simulink model "Bebop_sim_spline_without_joy"  (R2018a)
settings: Solver=VariableStepAuto  StartTime=0.0  StopTime=15  FixedStep=.05  MaxStep=1  MinStep=0.1  RelTol=200  AbsTol=200
values from neighbouring files (symbols this model uses):
  g = 9.81    [initialize_race_no_realtime.m]    (also in initialize_race_realtime.m; initialize_race_realtime_backup_cubic.m; moving_average_rls_own.m = P(i-1)*meas*(lambda+meas*P(i-1)*meas)^-1)
  gates = sim_gates(:,:,1)    [eval_sim.m]    (also in initialize_race_realtime.m = [dist,0,height,deg2rad(110); initialize_race_realtime_backup_cubic.m = [dist,0,height,deg2rad(110); plot_sim.m)
  max_rot_Z = (90)*pi/180    (= 1.57079632679)    [Bebop_sim_init.m]    (also in initialize_race_no_realtime.m = 1.0471975512; initialize_race_realtime.m; initialize_race_realtime_backup_cubic.m; run_batch1.m = list_agility(idx_agility)*max_rot_Z)
  max_theta_X = (40)*pi/180    (= 0.698131700798)    [Bebop_sim_init.m]    (also in initialize_race_no_realtime.m = 0.13962634016; initialize_race_realtime.m = 1.308996939; initialize_race_realtime_backup_cubic.m = 1.308996939; run_batch1.m = list_agility(idx_agility)*max_theta_X)
  max_theta_Y = (40)*pi/180    (= 0.698131700798)    [Bebop_sim_init.m]    (also in initialize_race_no_realtime.m = 0.13962634016; initialize_race_realtime.m = 1.308996939; initialize_race_realtime_backup_cubic.m = 1.308996939; run_batch1.m = list_agility(idx_agility)*max_theta_Y)
  max_v_Z = .5    (= 0.5)    [Bebop_sim_init.m]    (also in initialize_race_no_realtime.m = 1; initialize_race_realtime.m = 3; initialize_race_realtime_backup_cubic.m = 3; run_batch1.m = list_agility(idx_agility)*max_v_Z)
  splines = zeros(3,4,size(gates,1))    [initialize_race_no_realtime.m]    (also in show_splines.m)
libraries: simulink x4, sharedtransform x2, aerolibutil x1
settings Model: EnablePacing=on  Creator=vinni  LastModifiedBy=vinni
settings HardwareCC: ProdBitPerLong=64  ProdHWDeviceType=Intel->x86-64 (Linux 64)

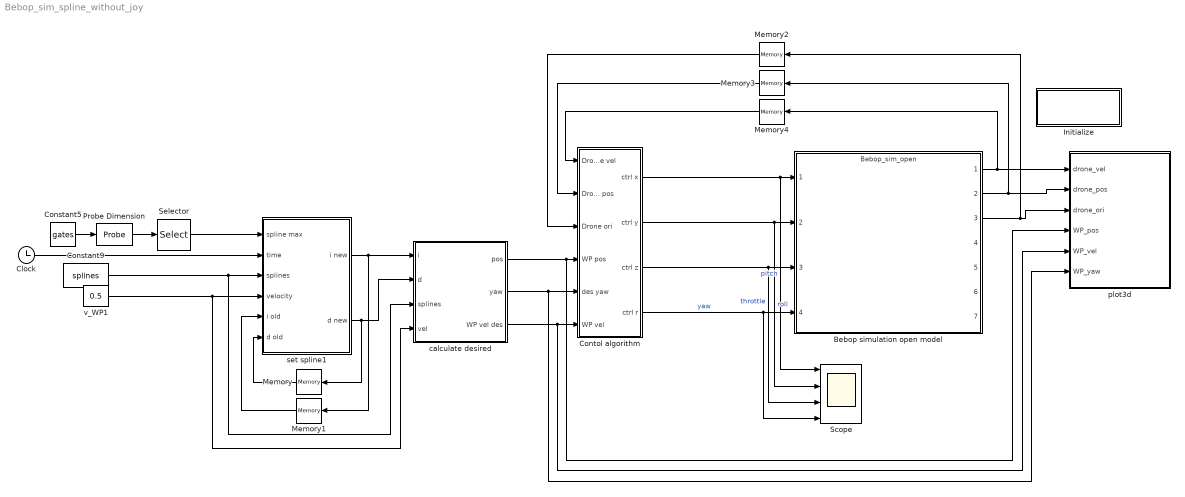
== system Bebop_sim_spline_without_joy ==
  Bebop simulation open model : ModelReference  ModelNameDialog=Bebop_sim_open.slx  SimulationMode=Normal  ModelReferenceVersion=1.31
  Clock : Clock
  Constant5 : Constant  Value=gates
  Constant9 : Constant  Value=splines
  Contol algorithm : Subsystem
  Initialize : Subsystem  TreatAsAtomicUnit=on
  Memory{,1..4} (5 alike) : Memory
  Probe Dimension : Probe  ProbeWidth=off  ProbeSampleTime=off  ProbeComplexSignal=off  ProbeSignalDimensions=on
  Scope : Scope  NumInputPorts=4
  Selector : Selector  IndexOptions=Index vector (dialog)  Indices=1  OutputSizes=1
  calculate desired : Subsystem
  plot3d : MATLAB Function  TreatAsAtomicUnit=on
  set spline1 : Subsystem
  v_WP1 : Constant  Value=0.5  VectorParams1D=off
  wires:
  Bebop simulation open model/2 -> Memory3/1, plot3d/2(drone_pos)
  Bebop simulation open model/3 -> Memory2/1, plot3d/3(drone_ori)
  Contol algorithm/2(ctrl y) -> Scope/2, Bebop simulation open model/2  "roll"
  Bebop simulation open model/1 -> Memory4/1, plot3d/1(drone_vel)
  Contol algorithm/1(ctrl x) -> Scope/1, Bebop simulation open model/1  "pitch"
  Contol algorithm/4(ctrl r) -> Scope/4, Bebop simulation open model/4  "yaw"
  Contol algorithm/3(ctrl z) -> Scope/3, Bebop simulation open model/3  "throttle"
  Constant9/1 -> set spline1/3(splines), calculate desired/3(splines)
  Selector/1 -> set spline1/1(spline max)
  Constant5/1 -> Probe Dimension/1
  Probe Dimension/1 -> Selector/1
  calculate desired/1(pos) -> Contol algorithm/4(WP pos), plot3d/4(WP_pos)
  Clock/1 -> set spline1/2(time)
  calculate desired/2(yaw) -> plot3d/6(WP_yaw), Contol algorithm/5(des yaw)
  calculate desired/3(WP vel des) -> plot3d/5(WP_vel), Contol algorithm/6(WP vel)
  set spline1/2(d new) -> Memory/1, calculate desired/2(d)
  Memory/1 -> set spline1/6(d old)
  set spline1/1(i new) -> Memory1/1, calculate desired/1(i)
  Memory1/1 -> set spline1/5(i old)
  v_WP1/1 -> set spline1/4(velocity), calculate desired/4(vel)
  Memory2/1 -> Contol algorithm/3(Drone ori)
  Memory3/1 -> Contol algorithm/2(Drone pos)
  Memory4/1 -> Contol algorithm/1(Drone vel)

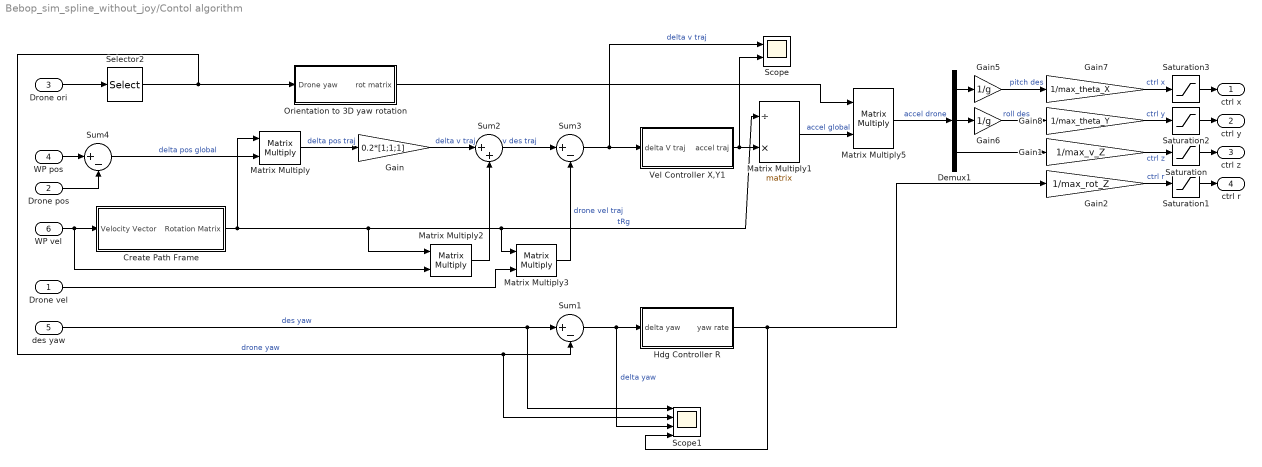
== system Bebop_sim_spline_without_joy/Contol algorithm ==
  Drone vel : Inport
  Drone pos : Inport  Port=2
  Drone ori : Inport  Port=3
  WP pos : Inport  Port=4
  des yaw : Inport  Port=5
  WP vel : Inport  Port=6
  Create Path Frame : Subsystem
  Demux1 : Demux  Outputs=3
  Gain : Gain  Gain=0.2*[1;1;1]
  Gain1 : Gain  Gain=1/max_v_Z
  Gain2 : Gain  Gain=1/max_rot_Z
  Gain5 : Gain  Gain=1/g
  Gain6 : Gain  Gain=1/g
  Gain7 : Gain  Gain=1/max_theta_X
  Gain8 : Gain  Gain=1/max_theta_Y
  Hdg Controller R : Subsystem
  Matrix Multiply{,2..3,5} (4 alike) : Product  Inputs=**  Multiplication=Matrix(*)
  Matrix Multiply1 : Product  Inputs=/*  Multiplication=Matrix(*)
  Orientation to 3D yaw rotation : Subsystem
  Saturation{,1..3} (4 alike) : Saturate  UpperLimit=1  LowerLimit=-1
  Scope : Scope  NumInputPorts=2
  Scope1 : Scope  NumInputPorts=4
  Selector2 : Selector  InputPortWidth=3  IndexOptions=Index vector (dialog)  Indices=3  OutputSizes=1
  Sum1 : Sum  Inputs=|+-
  Sum2 : Sum  Inputs=|++
  Sum3 : Sum  Inputs=|+-
  Sum4 : Sum  Inputs=|+-
  Vel Controller X,Y1 : Subsystem
  ctrl x : Outport
  ctrl y : Outport  Port=2
  ctrl z : Outport  Port=3
  ctrl r : Outport  Port=4
  wires:
  Sum4/1 -> Matrix Multiply/2  "delta pos global"
  Matrix Multiply/1 -> Gain/1  "delta pos traj"
  Create Path Frame/1(Rotation Matrix) -> Matrix Multiply/1, Matrix Multiply2/1, Matrix Multiply1/1, Matrix Multiply3/1  "tRg"
  WP vel/1 -> Matrix Multiply2/2, Create Path Frame/1(Velocity Vector)
  Drone pos/1 -> Sum4/2
  WP pos/1 -> Sum4/1
  Drone vel/1 -> Matrix Multiply3/2
  Gain/1 -> Sum2/1  "delta v traj"
  Drone ori/1 -> Selector2/1
  des yaw/1 -> Scope1/1, Sum1/1  "des yaw"
  Selector2/1 -> Scope1/2, Sum1/2, Orientation to 3D yaw rotation/1(Drone yaw)  "drone yaw"
  Sum1/1 -> Scope1/3, Hdg Controller R/1(delta yaw)  "delta yaw"
  Hdg Controller R/1(yaw rate) -> Scope1/4, Gain2/1
  Sum2/1 -> Sum3/1  "v des traj"
  Matrix Multiply2/1 -> Sum2/2
  Matrix Multiply3/1 -> Sum3/2  "drone vel traj"
  Sum3/1 -> Scope/1, Vel Controller X,Y1/1(delta V traj)  "delta v traj"
  Matrix Multiply1/1 -> Matrix Multiply5/2  "accel global"
  Vel Controller X,Y1/1(accel traj) -> Scope/2, Matrix Multiply1/2
  Orientation to 3D yaw rotation/1(rot matrix) -> Matrix Multiply5/1
  Matrix Multiply5/1 -> Demux1/1  "accel drone"
  Demux1/1 -> Gain5/1
  Demux1/2 -> Gain6/1
  Gain7/1 -> Saturation3/1  "ctrl x"
  Gain8/1 -> Saturation2/1  "ctrl y"
  Saturation2/1 -> ctrl y/1
  Gain5/1 -> Gain7/1  "pitch des"
  Gain6/1 -> Gain8/1  "roll des"
  Saturation3/1 -> ctrl x/1
  Gain1/1 -> Saturation/1  "ctrl z"
  Saturation/1 -> ctrl z/1
  Demux1/3 -> Gain1/1
  Gain2/1 -> Saturation1/1  "ctrl r"
  Saturation1/1 -> ctrl r/1

== system Bebop_sim_spline_without_joy/Initialize ==
  Event Listener : EventListener  DisableCoverage=on  EventName=reset
  reset_plot : MATLAB Function  TreatAsAtomicUnit=on

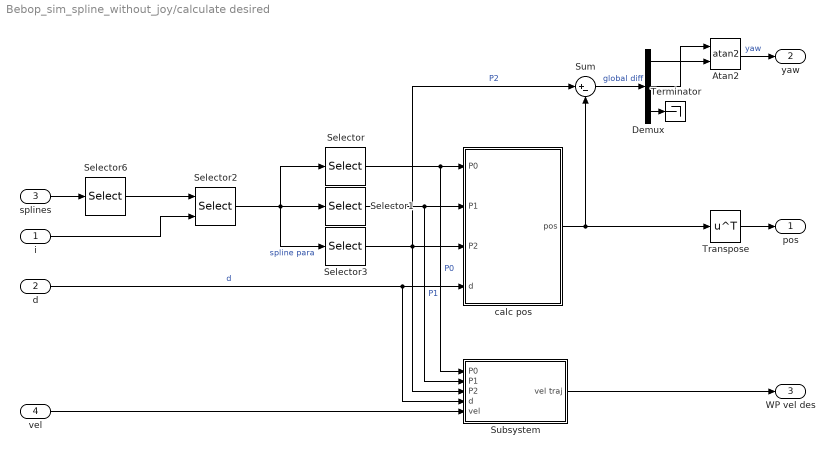
== system Bebop_sim_spline_without_joy/calculate desired ==
  i : Inport
  d : Inport  Port=2
  splines : Inport  Port=3
  vel : Inport  Port=4
  Atan2 : Trigonometry  Operator=atan2
  Demux : Demux  Outputs=3
  Selector : Selector  NumberOfDimensions=2  InputPortWidth=3  IndexOptions=Index vector (dialog),Select all  Indices=1,1  OutputSizes=1,1
  Selector1 : Selector  NumberOfDimensions=2  InputPortWidth=3  IndexOptions=Index vector (dialog),Select all  Indices=2,1  OutputSizes=1,1
  Selector2 : Selector  NumberOfDimensions=3  IndexMode=Zero-based  InputPortWidth=3  IndexOptions=Select all,Select all,Index vector (port)  Indices=3,1,1  OutputSizes=1,1,1
  Selector3 : Selector  NumberOfDimensions=2  InputPortWidth=3  IndexOptions=Index vector (dialog),Select all  Indices=3,1  OutputSizes=1,1
  Selector6 : Selector  NumberOfDimensions=3  InputPortWidth=3  IndexOptions=Select all,Index vector (dialog),Select all  Indices=3,[1,2,3],1  OutputSizes=1,1,1
  Subsystem : Subsystem
  Sum : Sum  Inputs=|+-
  Terminator : Terminator
  Transpose : Math  Operator=transpose  SaturateOnIntegerOverflow=on
  calc pos : Subsystem
  pos : Outport
  yaw : Outport  Port=2
  WP vel des : Outport  Port=3
  wires:
  splines/1 -> Selector6/1
  i/1 -> Selector2/2
  Selector2/1 -> Selector3/1, Selector1/1, Selector/1  "spline para"
  Selector/1 -> Subsystem/1(P0), calc pos/1(P0)  "P0"
  Selector1/1 -> Subsystem/2(P1), calc pos/2(P1)  "P1"
  Selector3/1 -> Sum/1, Subsystem/3(P2), calc pos/3(P2)  "P2"
  d/1 -> calc pos/4(d), Subsystem/4(d)  "d"
  calc pos/1(pos) -> Sum/2, Transpose/1
  Selector6/1 -> Selector2/1
  Sum/1 -> Demux/1  "global diff"
  Demux/2 -> Atan2/1
  Demux/1 -> Atan2/2
  Demux/3 -> Terminator/1
  Atan2/1 -> yaw/1  "yaw"
  vel/1 -> Subsystem/5(vel)
  Subsystem/1(vel traj) -> WP vel des/1
  Transpose/1 -> pos/1

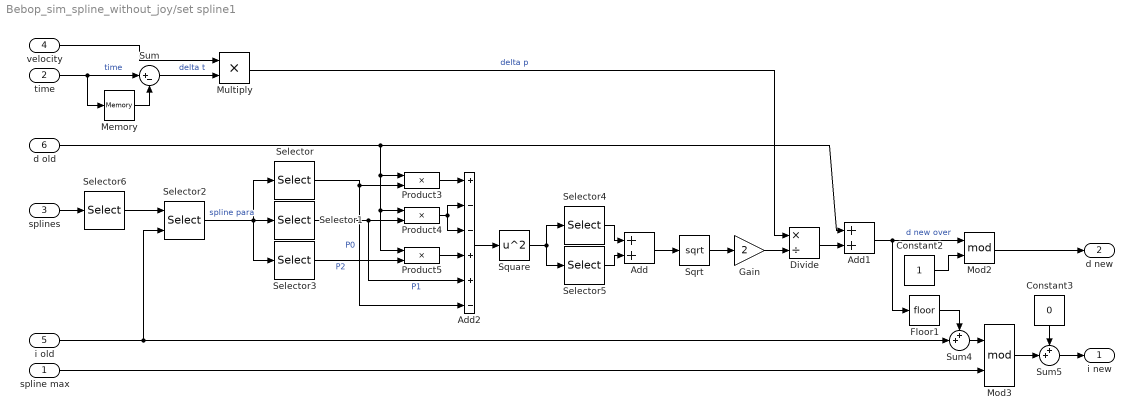
== system Bebop_sim_spline_without_joy/set spline1 ==
  spline max : Inport
  time : Inport  Port=2
  splines : Inport  Port=3
  velocity : Inport  Port=4
  i old : Inport  Port=5
  d old : Inport  Port=6
  Add : Sum
  Add1 : Sum
  Add2 : Sum  Inputs=+--++-
  Constant2 : Constant
  Constant3 : Constant  Value=0
  Divide : Product  Inputs=*/
  Floor1 : Rounding
  Gain : Gain  Gain=2
  Memory : Memory
  Mod2 : Math  Operator=mod  SaturateOnIntegerOverflow=on
  Mod3 : Math  Operator=mod  SaturateOnIntegerOverflow=on
  Multiply : Product
  Product3 : Product
  Product4 : Product
  Product5 : Product
  Selector : Selector  NumberOfDimensions=2  InputPortWidth=3  IndexOptions=Index vector (dialog),Select all  Indices=1,1  OutputSizes=1,1
  Selector1 : Selector  NumberOfDimensions=2  InputPortWidth=3  IndexOptions=Index vector (dialog),Select all  Indices=2,1  OutputSizes=1,1
  Selector2 : Selector  NumberOfDimensions=3  IndexMode=Zero-based  InputPortWidth=3  IndexOptions=Select all,Select all,Index vector (port)  Indices=3,1,1  OutputSizes=1,1,1
  Selector3 : Selector  NumberOfDimensions=2  InputPortWidth=3  IndexOptions=Index vector (dialog),Select all  Indices=3,1  OutputSizes=1,1
  Selector4 : Selector  InputPortWidth=3  IndexOptions=Index vector (dialog)  Indices=2  OutputSizes=1
  Selector5 : Selector  InputPortWidth=3  IndexOptions=Index vector (dialog)  Indices=1  OutputSizes=1
  Selector6 : Selector  NumberOfDimensions=3  InputPortWidth=3  IndexOptions=Select all,Index vector (dialog),Select all  Indices=3,[1,2,3],1  OutputSizes=1,1,1
  Sqrt : Sqrt  SaturateOnIntegerOverflow=on
  Square : Math  Operator=square  SaturateOnIntegerOverflow=on
  Sum : Sum  Inputs=|+-
  Sum4 : Sum  Inputs=++|
  Sum5 : Sum  Inputs=++|
  i new : Outport
  d new : Outport  Port=2
  wires:
  time/1 -> Sum/1, Memory/1  "time"
  Memory/1 -> Sum/2
  Sum/1 -> Multiply/2  "delta t"
  velocity/1 -> Multiply/1
  Multiply/1 -> Divide/1  "delta p"
  i old/1 -> Selector2/2, Sum4/2
  Selector1/1 -> Product4/2, Add2/5  "P1"
  Selector/1 -> Add2/6, Product3/2  "P0"
  splines/1 -> Selector6/1
  Selector6/1 -> Selector2/1
  Selector2/1 -> Selector/1, Selector3/1, Selector1/1  "spline para"
  Selector5/1 -> Add/2
  d old/1 -> Add1/1, Product5/1, Product4/1, Product3/1
  Add2/1 -> Square/1
  Selector4/1 -> Add/1
  Selector3/1 -> Product5/2  "P2"
  Product4/1 -> Add2/2, Add2/3
  Product3/1 -> Add2/1
  Product5/1 -> Add2/4
  Square/1 -> Selector5/1, Selector4/1
  Add/1 -> Sqrt/1
  Sqrt/1 -> Gain/1
  Gain/1 -> Divide/2
  Divide/1 -> Add1/2
  spline max/1 -> Mod3/2
  Constant2/1 -> Mod2/2
  Mod2/1 -> d new/1
  Add1/1 -> Mod2/1, Floor1/1  "d new over"
  Floor1/1 -> Sum4/1
  Sum4/1 -> Mod3/1
  Mod3/1 -> Sum5/2
  Constant3/1 -> Sum5/1
  Sum5/1 -> i new/1

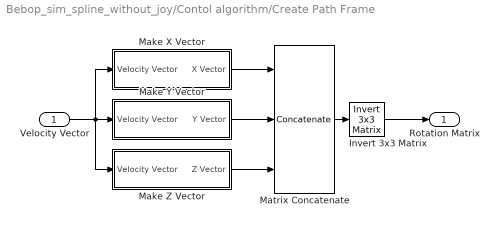
== system Bebop_sim_spline_without_joy/Contol algorithm/Create Path Frame ==
  Velocity Vector : Inport
  Invert 3x3 Matrix : aerolibutil/Invert  3x3 Matrix
  Make X Vector : Subsystem
  Make Y Vector : Subsystem
  Make Z Vector : Subsystem
  Matrix Concatenate : Concatenate  NumInputs=3  Mode=Multidimensional array  ConcatenateDimension=2
  Rotation Matrix : Outport
  wires:
  Velocity Vector/1 -> Make Z Vector/1(Velocity Vector), Make X Vector/1(Velocity Vector), Make Y Vector/1(Velocity Vector)
  Make Y Vector/1(Y Vector) -> Matrix Concatenate/2
  Make X Vector/1(X Vector) -> Matrix Concatenate/1
  Make Z Vector/1(Z Vector) -> Matrix Concatenate/3
  Matrix Concatenate/1 -> Invert 3x3 Matrix/1
  Invert 3x3 Matrix/1 -> Rotation Matrix/1

== system Bebop_sim_spline_without_joy/Contol algorithm/Hdg Controller R ==
  delta yaw : Inport
  Atan2 : Trigonometry  Operator=atan2
  Cos : Trigonometry  Operator=sincos
  PID Controller : simulink/Continuous/PID Controller  Controller=PID  TimeDomain=Continuous-time  SampleTime=-1  IntegratorMethod=Forward Euler  FilterMethod=Forward Euler  Form=Parallel  UseFilter=on  ControllerParametersSource=internal  P=3  I=0.5  D=0  N=10  InitialConditionSource=internal  InitialConditionForIntegrator=0  InitialConditionForFilter=0  ExternalReset=none  LimitOutput=off  UpperSaturationLimit=inf  LowerSaturationLimit=-inf  LinearizeAsGain=on  AntiWindupMode=none  Kb=1  TrackingMode=off  Kt=1  PParamMin=[]  PParamMax=[]  IParamMin=[]  IParamMax=[]  DParamMin=[]  DParamMax=[]  NParamMin=[]  NParamMax=[]  KbParamMin=[]  KbParamMax=[]  KtParamMin=[]  KtParamMax=[]  POutMin=[]  POutMax=[]  IOutMin=[]  IOutMax=[]  DOutMin=[]  DOutMax=[]  NOutMin=[]  NOutMax=[]  KbOutMin=[]  KbOutMax=[]  KtOutMin=[]  KtOutMax=[]  IntegratorOutMin=[]  IntegratorOutMax=[]  FilterOutMin=[]  FilterOutMax=[]  SumOutMin=[]  SumOutMax=[]  SumI1OutMin=[]  SumI1OutMax=[]  SumI2OutMin=[]  SumI2OutMax=[]  SumI3OutMin=[]  SumI3OutMax=[]  SumDOutMin=[]  SumDOutMax=[]  SaturationOutMin=[]  SaturationOutMax=[]  IntegratorContinuousStateAttributes=''  IntegratorStateMustResolveToSignalObject=off  IntegratorRTWStateStorageClass=Auto  FilterContinuousStateAttributes=''  FilterStateMustResolveToSignalObject=off  FilterRTWStateStorageClass=Auto  DifferentiatorICPrevScaledInput=0  DifferentiatorOutMin=[]  DifferentiatorOutMax=[]  FilterDiffOutCoefMin=[]  FilterDiffOutCoefMax=[]  SumDenOutMin=[]  SumDenOutMax=[]  SumNumOutMin=[]  SumNumOutMax=[]  ReciprocalOutMin=[]  ReciprocalOutMax=[]  DivideOutMin=[]  DivideOutMax=[]  TunerSelectOption=Transfer Function Based (PID Tuner App)
  yaw rate : Outport
  wires:
  delta yaw/1 -> Cos/1  "delta yaw"
  Cos/1 -> Atan2/1
  PID Controller/1 -> yaw rate/1  "yaw rate"
  Atan2/1 -> PID Controller/1  "d yaw"
  Cos/2 -> Atan2/2

== system Bebop_sim_spline_without_joy/Contol algorithm/Orientation to 3D yaw rotation ==
  Drone yaw : Inport
  Constant1 : Constant  Value=0
  Rotation Angles to Direction Cosine Matrix : sharedtransform/Rotation Angles to Direction Cosine Matrix  rotationOrder=ZYX  aMode=aMode
      settings: SourceProductBaseCode=AE
  Vector Concatenate : Concatenate  NumInputs=3
  rot matrix : Outport
  wires:
  Constant1/1 -> Vector Concatenate/2, Vector Concatenate/3
  Vector Concatenate/1 -> Rotation Angles to Direction Cosine Matrix/1
  Drone yaw/1 -> Vector Concatenate/1  "yaw"
  Rotation Angles to Direction Cosine Matrix/1 -> rot matrix/1  "rot matrix"

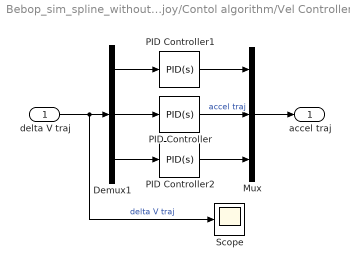
== system Bebop_sim_spline_without_joy/Contol algorithm/Vel Controller X,Y1 ==
  delta V traj : Inport
  Demux1 : Demux  Outputs=3
  Mux : Mux  Inputs=3
  PID Controller : simulink/Continuous/PID Controller  Controller=PID  TimeDomain=Continuous-time  SampleTime=-1  IntegratorMethod=Forward Euler  FilterMethod=Forward Euler  Form=Parallel  UseFilter=on  ControllerParametersSource=internal  P=4  I=2.5  D=0  N=10  InitialConditionSource=internal  InitialConditionForIntegrator=0  InitialConditionForFilter=0  ExternalReset=none  LimitOutput=off  UpperSaturationLimit=inf  LowerSaturationLimit=-inf  LinearizeAsGain=on  AntiWindupMode=none  Kb=1  TrackingMode=off  Kt=1  PParamMin=[]  PParamMax=[]  IParamMin=[]  IParamMax=[]  DParamMin=[]  DParamMax=[]  NParamMin=[]  NParamMax=[]  KbParamMin=[]  KbParamMax=[]  KtParamMin=[]  KtParamMax=[]  POutMin=[]  POutMax=[]  IOutMin=[]  IOutMax=[]  DOutMin=[]  DOutMax=[]  NOutMin=[]  NOutMax=[]  KbOutMin=[]  KbOutMax=[]  KtOutMin=[]  KtOutMax=[]  IntegratorOutMin=[]  IntegratorOutMax=[]  FilterOutMin=[]  FilterOutMax=[]  SumOutMin=[]  SumOutMax=[]  SumI1OutMin=[]  SumI1OutMax=[]  SumI2OutMin=[]  SumI2OutMax=[]  SumI3OutMin=[]  SumI3OutMax=[]  SumDOutMin=[]  SumDOutMax=[]  SaturationOutMin=[]  SaturationOutMax=[]  IntegratorContinuousStateAttributes=''  IntegratorStateMustResolveToSignalObject=off  IntegratorRTWStateStorageClass=Auto  FilterContinuousStateAttributes=''  FilterStateMustResolveToSignalObject=off  FilterRTWStateStorageClass=Auto  DifferentiatorICPrevScaledInput=0  DifferentiatorOutMin=[]  DifferentiatorOutMax=[]  FilterDiffOutCoefMin=[]  FilterDiffOutCoefMax=[]  SumDenOutMin=[]  SumDenOutMax=[]  SumNumOutMin=[]  SumNumOutMax=[]  ReciprocalOutMin=[]  ReciprocalOutMax=[]  DivideOutMin=[]  DivideOutMax=[]  TunerSelectOption=Transfer Function Based (PID Tuner App)
  PID Controller1 : simulink/Continuous/PID Controller  Controller=PID  TimeDomain=Continuous-time  SampleTime=-1  IntegratorMethod=Forward Euler  FilterMethod=Forward Euler  Form=Parallel  UseFilter=on  ControllerParametersSource=internal  P=4  I=2  D=0  N=10  InitialConditionSource=internal  InitialConditionForIntegrator=0  InitialConditionForFilter=0  ExternalReset=none  LimitOutput=off  UpperSaturationLimit=inf  LowerSaturationLimit=-inf  LinearizeAsGain=on  AntiWindupMode=none  Kb=1  TrackingMode=off  Kt=1  PParamMin=[]  PParamMax=[]  IParamMin=[]  IParamMax=[]  DParamMin=[]  DParamMax=[]  NParamMin=[]  NParamMax=[]  KbParamMin=[]  KbParamMax=[]  KtParamMin=[]  KtParamMax=[]  POutMin=[]  POutMax=[]  IOutMin=[]  IOutMax=[]  DOutMin=[]  DOutMax=[]  NOutMin=[]  NOutMax=[]  KbOutMin=[]  KbOutMax=[]  KtOutMin=[]  KtOutMax=[]  IntegratorOutMin=[]  IntegratorOutMax=[]  FilterOutMin=[]  FilterOutMax=[]  SumOutMin=[]  SumOutMax=[]  SumI1OutMin=[]  SumI1OutMax=[]  SumI2OutMin=[]  SumI2OutMax=[]  SumI3OutMin=[]  SumI3OutMax=[]  SumDOutMin=[]  SumDOutMax=[]  SaturationOutMin=[]  SaturationOutMax=[]  IntegratorContinuousStateAttributes=''  IntegratorStateMustResolveToSignalObject=off  IntegratorRTWStateStorageClass=Auto  FilterContinuousStateAttributes=''  FilterStateMustResolveToSignalObject=off  FilterRTWStateStorageClass=Auto  DifferentiatorICPrevScaledInput=0  DifferentiatorOutMin=[]  DifferentiatorOutMax=[]  FilterDiffOutCoefMin=[]  FilterDiffOutCoefMax=[]  SumDenOutMin=[]  SumDenOutMax=[]  SumNumOutMin=[]  SumNumOutMax=[]  ReciprocalOutMin=[]  ReciprocalOutMax=[]  DivideOutMin=[]  DivideOutMax=[]  TunerSelectOption=Transfer Function Based (PID Tuner App)
  PID Controller2 : simulink/Continuous/PID Controller  Controller=PID  TimeDomain=Continuous-time  SampleTime=-1  IntegratorMethod=Forward Euler  FilterMethod=Forward Euler  Form=Parallel  UseFilter=on  ControllerParametersSource=internal  P=1  I=3  D=0  N=10  InitialConditionSource=internal  InitialConditionForIntegrator=0  InitialConditionForFilter=0  ExternalReset=none  LimitOutput=off  UpperSaturationLimit=inf  LowerSaturationLimit=-inf  LinearizeAsGain=on  AntiWindupMode=none  Kb=1  TrackingMode=off  Kt=1  PParamMin=[]  PParamMax=[]  IParamMin=[]  IParamMax=[]  DParamMin=[]  DParamMax=[]  NParamMin=[]  NParamMax=[]  KbParamMin=[]  KbParamMax=[]  KtParamMin=[]  KtParamMax=[]  POutMin=[]  POutMax=[]  IOutMin=[]  IOutMax=[]  DOutMin=[]  DOutMax=[]  NOutMin=[]  NOutMax=[]  KbOutMin=[]  KbOutMax=[]  KtOutMin=[]  KtOutMax=[]  IntegratorOutMin=[]  IntegratorOutMax=[]  FilterOutMin=[]  FilterOutMax=[]  SumOutMin=[]  SumOutMax=[]  SumI1OutMin=[]  SumI1OutMax=[]  SumI2OutMin=[]  SumI2OutMax=[]  SumI3OutMin=[]  SumI3OutMax=[]  SumDOutMin=[]  SumDOutMax=[]  SaturationOutMin=[]  SaturationOutMax=[]  IntegratorContinuousStateAttributes=''  IntegratorStateMustResolveToSignalObject=off  IntegratorRTWStateStorageClass=Auto  FilterContinuousStateAttributes=''  FilterStateMustResolveToSignalObject=off  FilterRTWStateStorageClass=Auto  DifferentiatorICPrevScaledInput=0  DifferentiatorOutMin=[]  DifferentiatorOutMax=[]  FilterDiffOutCoefMin=[]  FilterDiffOutCoefMax=[]  SumDenOutMin=[]  SumDenOutMax=[]  SumNumOutMin=[]  SumNumOutMax=[]  ReciprocalOutMin=[]  ReciprocalOutMax=[]  DivideOutMin=[]  DivideOutMax=[]  TunerSelectOption=Transfer Function Based (PID Tuner App)
  Scope : Scope
  accel traj : Outport
  wires:
  delta V traj/1 -> Scope/1, Demux1/1  "delta V traj"
  PID Controller/1 -> Mux/2  "accel traj"
  Demux1/1 -> PID Controller1/1
  Demux1/2 -> PID Controller/1
  Demux1/3 -> PID Controller2/1
  PID Controller2/1 -> Mux/3
  PID Controller1/1 -> Mux/1
  Mux/1 -> accel traj/1

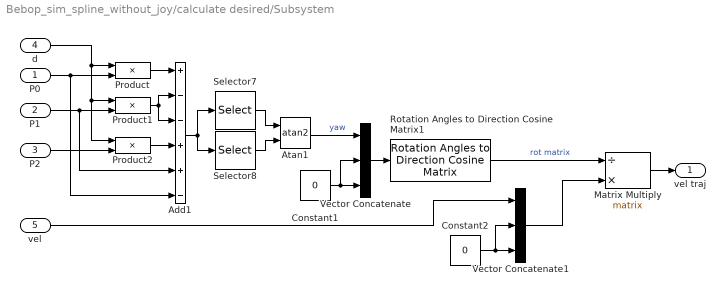
== system Bebop_sim_spline_without_joy/calculate desired/Subsystem ==
  P0 : Inport
  P1 : Inport  Port=2
  P2 : Inport  Port=3
  d : Inport  Port=4
  vel : Inport  Port=5
  Add1 : Sum  Inputs=+--++-
  Atan1 : Trigonometry  Operator=atan2
  Constant1 : Constant  Value=0
  Constant2 : Constant  Value=0
  Matrix Multiply : Product  Inputs=/*  Multiplication=Matrix(*)
  Product : Product
  Product1 : Product
  Product2 : Product
  Rotation Angles to Direction Cosine Matrix1 : sharedtransform/Rotation Angles to Direction Cosine Matrix  rotationOrder=ZYX  aMode=aMode
      settings: SourceProductBaseCode=AE
  Selector7 : Selector  InputPortWidth=3  IndexOptions=Index vector (dialog)  Indices=2  OutputSizes=1
  Selector8 : Selector  InputPortWidth=3  IndexOptions=Index vector (dialog)  Indices=1  OutputSizes=1
  Vector Concatenate : Concatenate  NumInputs=3
  Vector Concatenate1 : Concatenate  NumInputs=3
  vel traj : Outport
  wires:
  Product2/1 -> Add1/4
  Product1/1 -> Add1/3, Add1/2
  Product/1 -> Add1/1
  Atan1/1 -> Vector Concatenate/1  "yaw"
  Selector7/1 -> Atan1/1
  Constant1/1 -> Vector Concatenate/2, Vector Concatenate/3
  Vector Concatenate1/1 -> Matrix Multiply/2
  P2/1 -> Product2/2
  Matrix Multiply/1 -> vel traj/1
  Vector Concatenate/1 -> Rotation Angles to Direction Cosine Matrix1/1
  P1/1 -> Add1/5, Product1/2
  P0/1 -> Add1/6, Product/2
  d/1 -> Product2/1, Product1/1, Product/1
  Constant2/1 -> Vector Concatenate1/2, Vector Concatenate1/3
  vel/1 -> Vector Concatenate1/1
  Rotation Angles to Direction Cosine Matrix1/1 -> Matrix Multiply/1  "rot matrix"
  Add1/1 -> Selector8/1, Selector7/1
  Selector8/1 -> Atan1/2

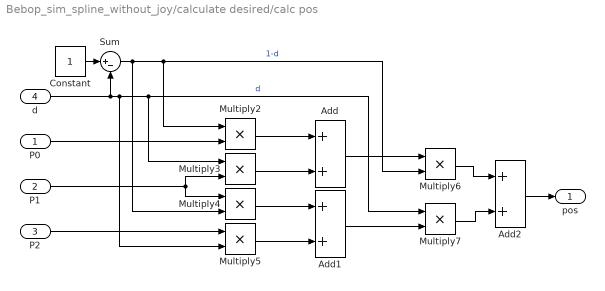
== system Bebop_sim_spline_without_joy/calculate desired/calc pos ==
  P0 : Inport
  P1 : Inport  Port=2
  P2 : Inport  Port=3
  d : Inport  Port=4
  Add : Sum
  Add1 : Sum
  Add2 : Sum
  Constant : Constant
  Multiply{2..7} (6 alike) : Product
  Sum : Sum  Inputs=|+-
  pos : Outport
  wires:
  d/1 -> Multiply5/2, Multiply7/1, Multiply3/1, Sum/2  "d"
  Sum/1 -> Multiply4/2, Multiply6/2, Multiply2/1  "1-d"
  Constant/1 -> Sum/1
  P0/1 -> Multiply2/2
  P1/1 -> Multiply4/1, Multiply3/2
  P2/1 -> Multiply5/1
  Multiply3/1 -> Add/2
  Multiply2/1 -> Add/1
  Multiply4/1 -> Add1/1
  Multiply5/1 -> Add1/2
  Add/1 -> Multiply6/1
  Add1/1 -> Multiply7/2
  Multiply6/1 -> Add2/1
  Multiply7/1 -> Add2/2
  Add2/1 -> pos/1

== system Bebop_sim_spline_without_joy/Contol algorithm/Create Path Frame/Make X Vector ==
  Velocity Vector : Inport
  Make Unit : Subsystem
  X Vector : Outport
  wires:
  Velocity Vector/1 -> Make Unit/1(Vector)
  Make Unit/1(Unit Vector) -> X Vector/1

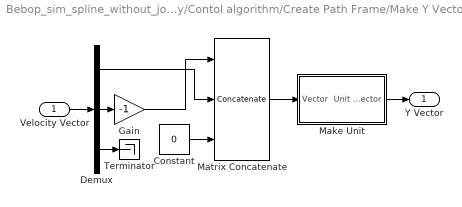
== system Bebop_sim_spline_without_joy/Contol algorithm/Create Path Frame/Make Y Vector ==
  Velocity Vector : Inport
  Constant : Constant  Value=0
  Demux : Demux  Outputs=3
  Gain : Gain  Gain=-1
  Make Unit : Subsystem
  Matrix Concatenate : Concatenate  NumInputs=3  Mode=Multidimensional array
  Terminator : Terminator
  Y Vector : Outport
  wires:
  Make Unit/1(Unit Vector) -> Y Vector/1
  Velocity Vector/1 -> Demux/1
  Demux/3 -> Terminator/1
  Demux/2 -> Gain/1
  Gain/1 -> Matrix Concatenate/1
  Demux/1 -> Matrix Concatenate/2
  Constant/1 -> Matrix Concatenate/3
  Matrix Concatenate/1 -> Make Unit/1(Vector)

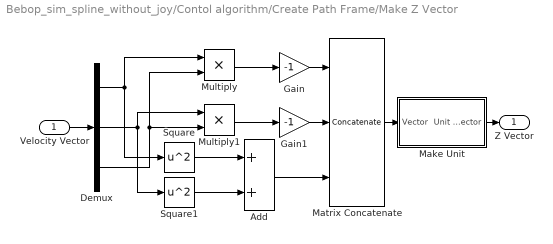
== system Bebop_sim_spline_without_joy/Contol algorithm/Create Path Frame/Make Z Vector ==
  Velocity Vector : Inport
  Add : Sum
  Demux : Demux  Outputs=3
  Gain : Gain  Gain=-1
  Gain1 : Gain  Gain=-1
  Make Unit : Subsystem
  Matrix Concatenate : Concatenate  NumInputs=3  Mode=Multidimensional array
  Multiply : Product
  Multiply1 : Product
  Square : Math  Operator=square  SaturateOnIntegerOverflow=on
  Square1 : Math  Operator=square  SaturateOnIntegerOverflow=on
  Z Vector : Outport
  wires:
  Make Unit/1(Unit Vector) -> Z Vector/1
  Velocity Vector/1 -> Demux/1
  Demux/3 -> Multiply/2, Multiply1/2
  Matrix Concatenate/1 -> Make Unit/1(Vector)
  Multiply/1 -> Gain/1
  Gain/1 -> Matrix Concatenate/1
  Demux/1 -> Square/1, Multiply/1
  Multiply1/1 -> Gain1/1
  Gain1/1 -> Matrix Concatenate/2
  Demux/2 -> Square1/1, Multiply1/1
  Add/1 -> Matrix Concatenate/3
  Square/1 -> Add/1
  Square1/1 -> Add/2

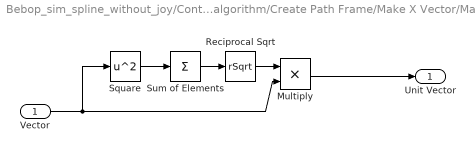
== system Bebop_sim_spline_without_joy/Contol algorithm/Create Path Frame/Make X Vector/Make Unit ==
  Vector : Inport
  Multiply : Product
  Reciprocal Sqrt : Sqrt  Operator=rSqrt  SaturateOnIntegerOverflow=on
  Square : Math  Operator=square  SaturateOnIntegerOverflow=on
  Sum of Elements : Sum  Inputs=+
  Unit Vector : Outport
  wires:
  Reciprocal Sqrt/1 -> Multiply/1
  Vector/1 -> Square/1, Multiply/2
  Square/1 -> Sum of Elements/1
  Multiply/1 -> Unit Vector/1
  Sum of Elements/1 -> Reciprocal Sqrt/1

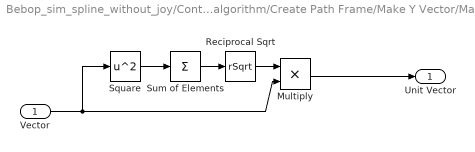
== system Bebop_sim_spline_without_joy/Contol algorithm/Create Path Frame/Make Y Vector/Make Unit ==
  Vector : Inport
  Multiply : Product
  Reciprocal Sqrt : Sqrt  Operator=rSqrt  SaturateOnIntegerOverflow=on
  Square : Math  Operator=square  SaturateOnIntegerOverflow=on
  Sum of Elements : Sum  Inputs=+
  Unit Vector : Outport
  wires:
  Reciprocal Sqrt/1 -> Multiply/1
  Vector/1 -> Square/1, Multiply/2
  Square/1 -> Sum of Elements/1
  Multiply/1 -> Unit Vector/1
  Sum of Elements/1 -> Reciprocal Sqrt/1

== system Bebop_sim_spline_without_joy/Contol algorithm/Create Path Frame/Make Z Vector/Make Unit ==
  Vector : Inport
  Multiply : Product
  Reciprocal Sqrt : Sqrt  Operator=rSqrt  SaturateOnIntegerOverflow=on
  Square : Math  Operator=square  SaturateOnIntegerOverflow=on
  Sum of Elements : Sum  Inputs=+
  Unit Vector : Outport
  wires:
  Reciprocal Sqrt/1 -> Multiply/1
  Vector/1 -> Square/1, Multiply/2
  Square/1 -> Sum of Elements/1
  Multiply/1 -> Unit Vector/1
  Sum of Elements/1 -> Reciprocal Sqrt/1

== matlab function Bebop_sim_spline_without_joy/plot3d ==
  data: drone_vel input; drone_pos input; drone_ori input; WP_pos input; WP_vel input; WP_yaw input
function plot3d(drone_vel, drone_pos, drone_ori, WP_pos, WP_vel, WP_yaw)
coder.extrinsic('delete')

children = get(gca, 'children');
delete(children(1:7));

gRb = eul2rotm([drone_ori(3),drone_ori(2),drone_ori(1)]);
length = 1;
x_bebop = gRb*[length;0;0];
y_bebop = gRb*[0;length;0];
z_bebop = gRb*[0;0;length];


plot3(drone_pos(1),drone_pos(2),drone_pos(3),'m.','MarkerSize',7)
plot3(drone_pos(1),drone_pos(2),0,'k.','MarkerSize',5)

plot3(drone_pos(1)+[0 drone_vel(1)],drone_pos(2)+[0 drone_vel(2)],drone_pos(3)+[0 drone_vel(3)],'k-','LineWidth',2)

plot3(drone_pos(1)+[0 x_bebop(1)],drone_pos(2)+[0 x_bebop(2)],drone_pos(3)+[0 x_bebop(3)],'r-')
plot3(drone_pos(1)+[0 y_bebop(1)],drone_pos(2)+[0 y_bebop(2)],drone_pos(3)+[0 y_bebop(3)],'g-')
plot3(drone_pos(1)+[0 z_bebop(1)],drone_pos(2)+[0 z_bebop(2)],drone_pos(3)+[0 z_bebop(3)],'b-')

plot3(WP_pos(1),WP_pos(2),WP_pos(3),'bx','MarkerSize',10)
plot3(WP_pos(1)+[0 WP_vel(1)],WP_pos(2)+[0 WP_vel(2)],WP_pos(3)+[0 WP_vel(3)],'b-','LineWidth',2)
plot3(WP_pos(1)+[0 cos(WP_yaw)],WP_pos(2)+[0 sin(WP_yaw)],WP_pos(3)+[0 0],'r-','LineWidth',1)

== matlab function Bebop_sim_spline_without_joy/Initialize/reset_plot ==
function reset_plot()
close all;
figure('units','normalized','outerposition',[0 0 0.5 1])
hold on
grid on
axis equal

for i=1:7
    plot3(0,0,0,'m.')
end

% axis([-5,5,-5,5,-2,2])
axis([-5,5,-5,5,0,4])
%view(-20,40) % 3D view
view(-90,90) % top view
%view(-90,0) % front view
xlabel('x')
ylabel('y')
zlabel('z')
